simulink model "myEmagModel"  (R2020a)
settings: Solver=VariableStepAuto  StartTime=0.0  StopTime=5  RelTol=1e-3
undefined symbols (not defined in the file): k1, k2, k3, Ki, Ks, L, m1, m2, m3, R, u_0, x_0
settings Model: Creator=tanzc  LastModifiedBy=tanzc
settings DataIOCC: ReturnWorkspaceOutputs=off

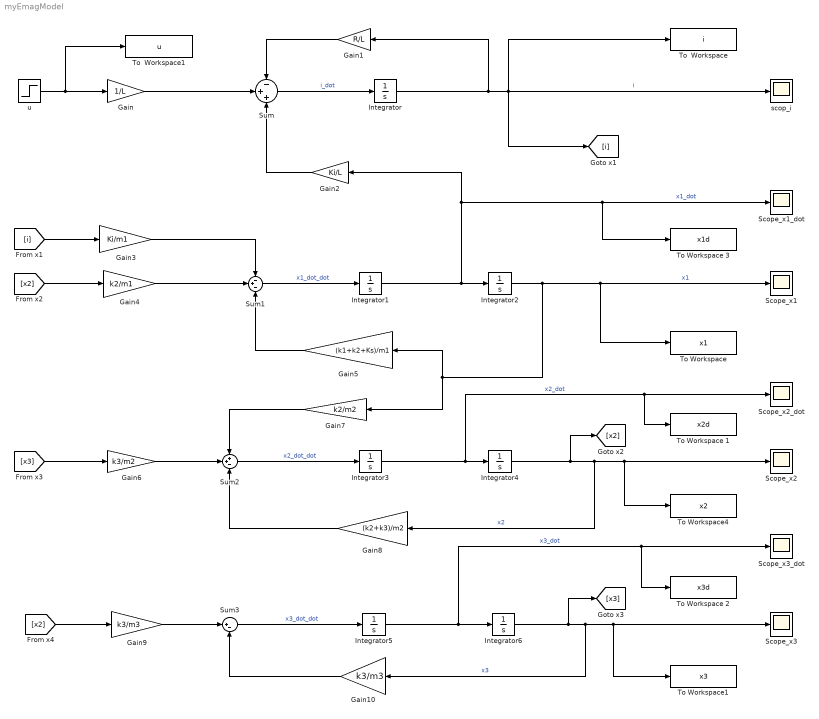
== system myEmagModel ==
  Gain : Gain  Gain=1/L
  Gain1 : Gain  Gain=R/L
  Gain10 : Gain  Gain=k3/m3
  Gain2 : Gain  Gain=Ki/L
  Gain3 : Gain  Gain=Ki/m1
  Gain4 : Gain  Gain=k2/m1
  Gain5 : Gain  Gain=(k1+k2+Ks)/m1
  Gain6 : Gain  Gain=k3/m2
  Gain7 : Gain  Gain=k2/m2
  Gain8 : Gain  Gain=(k2+k3)/m2
  Gain9 : Gain  Gain=k3/m3
  Integrator : Integrator  InitialCondition=x_0(1)
  Integrator1 : Integrator  InitialCondition=x_0(3)
  Integrator2 : Integrator  InitialCondition=x_0(2)
  Integrator3 : Integrator  InitialCondition=x_0(5)
  Integrator4 : Integrator  InitialCondition=x_0(4)
  Integrator5 : Integrator  InitialCondition=x_0(7)
  Integrator6 : Integrator  InitialCondition=x_0(6)
  Scope_x1 : Scope
  Scope_x1_dot : Scope
  Scope_x2 : Scope
  Scope_x2_dot : Scope
  Scope_x3 : Scope
  Scope_x3_dot : Scope
  Sum : Sum  Inputs=-++
  Sum1 : Sum  Inputs=-+-
  Sum2 : Sum  Inputs=++-
  Sum3 : Sum  Inputs=|+-
  To  Workspace : ToWorkspace  VariableName=i  SaveFormat=Structure With Time  SampleTime=-1
  To  Workspace1 : ToWorkspace  VariableName=u  SaveFormat=Structure With Time  SampleTime=-1
  "To Workspace " : ToWorkspace  VariableName=x1  SaveFormat=Structure With Time  SampleTime=-1
  To Workspace 1 : ToWorkspace  VariableName=x2d  SaveFormat=Structure With Time  SampleTime=-1
  To Workspace 2 : ToWorkspace  VariableName=x3d  SaveFormat=Structure With Time  SampleTime=-1
  To Workspace 3 : ToWorkspace  VariableName=x1d  SaveFormat=Structure With Time  SampleTime=-1
  To Workspace1 : ToWorkspace  VariableName=x3  SaveFormat=Structure With Time  SampleTime=-1
  To Workspace4 : ToWorkspace  VariableName=x2  SaveFormat=Structure With Time  SampleTime=-1
  scop_i : Scope
  u : Step  After=u_0  SampleTime=0
  wires:
  Integrator/1 -> Gain1/1, To  Workspace/1, scop_i/1, [i]  "i"
  Sum/1 -> Integrator/1  "i_dot"
  u/1 -> Gain/1, To  Workspace1/1
  Gain1/1 -> Sum/1
  Gain/1 -> Sum/2
  Gain2/1 -> Sum/3
  Integrator1/1 -> Integrator2/1, To Workspace 3/1, Scope_x1_dot/1, Gain2/1  "x1_dot"
  Sum1/1 -> Integrator1/1  "x1_dot_dot"
  [i] -> Gain3/1
  Gain3/1 -> Sum1/1
  [x2] -> Gain4/1
  Gain4/1 -> Sum1/2
  Integrator2/1 -> "To Workspace "/1, Scope_x1/1, Gain7/1, Gain5/1  "x1"
  Gain5/1 -> Sum1/3
  Integrator3/1 -> To Workspace 1/1, Scope_x2_dot/1, Integrator4/1  "x2_dot"
  Integrator4/1 -> To Workspace4/1, Scope_x2/1, Gain8/1, [x2]  "x2"
  Sum2/1 -> Integrator3/1  "x2_dot_dot"
  [x3] -> Gain6/1
  Gain6/1 -> Sum2/2
  Gain7/1 -> Sum2/1
  Gain8/1 -> Sum2/3
  Integrator5/1 -> To Workspace 2/1, Scope_x3_dot/1, Integrator6/1  "x3_dot"
  Sum3/1 -> Integrator5/1  "x3_dot_dot"
  Integrator6/1 -> To Workspace1/1, Scope_x3/1, Gain10/1, [x3]  "x3"
  Gain9/1 -> Sum3/1
  [x2] -> Gain9/1
  Gain10/1 -> Sum3/2
